simulink model "sis_segundo_orden_comparacion"  (R2018a)
settings: Solver=VariableStepAuto  StartTime=0.0  StopTime=10.0  RelTol=1e-3
settings Model: Creator=LENOVO  LastModifiedBy=LENOVO

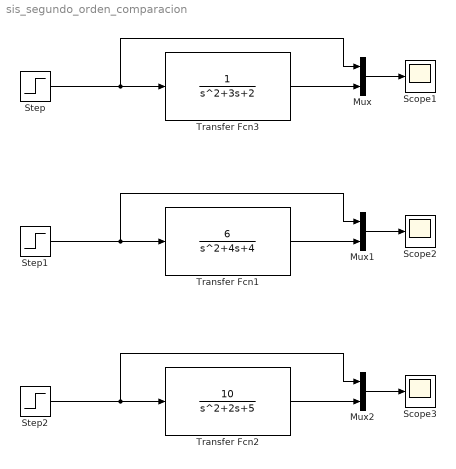
== system sis_segundo_orden_comparacion ==
  Mux : Mux  Inputs=2
  Mux1 : Mux  Inputs=2
  Mux2 : Mux  Inputs=2
  Scope1 : Scope
  Scope2 : Scope
  Scope3 : Scope
  Step : Step  SampleTime=0
  Step1 : Step  SampleTime=0
  Step2 : Step  SampleTime=0
  Transfer Fcn1 : TransferFcn  Numerator=[6]  Denominator=[1 4 4]
  Transfer Fcn2 : TransferFcn  Numerator=[10]  Denominator=[1 2 5]
  Transfer Fcn3 : TransferFcn  Denominator=[1 3 2]
  wires:
  Step/1 -> Mux/1, Transfer Fcn3/1
  Mux/1 -> Scope1/1
  Transfer Fcn3/1 -> Mux/2
  Step1/1 -> Mux1/1, Transfer Fcn1/1
  Transfer Fcn1/1 -> Mux1/2
  Mux1/1 -> Scope2/1
  Step2/1 -> Mux2/1, Transfer Fcn2/1
  Transfer Fcn2/1 -> Mux2/2
  Mux2/1 -> Scope3/1
